simulink model "buffer"  (R2020a)
settings: Solver=VariableStepAuto  StartTime=0.0  StopTime=10.0  RelTol=1e-3
settings Model: Creator=ysz  LastModifiedBy=ysz

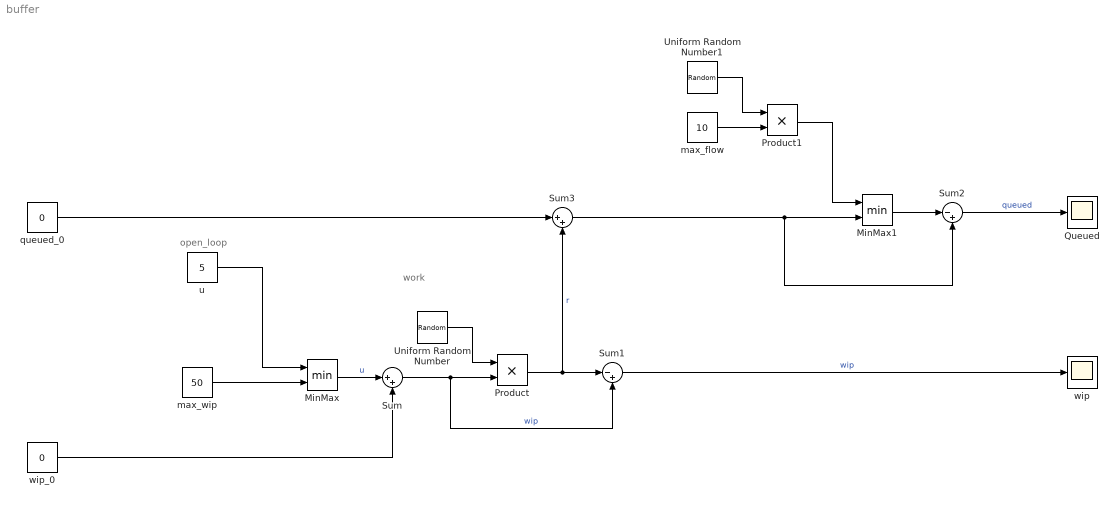
== system buffer ==
  note: open_loop
  note: work
  MinMax : MinMax  Inputs=2
  MinMax1 : MinMax  Inputs=2
  Product : Product
  Product1 : Product
  Queued : Scope
  Sum : Sum  Inputs=|++
  Sum1 : Sum  Inputs=|-+
  Sum2 : Sum  Inputs=|-+
  Sum3 : Sum  Inputs=|++
  Uniform Random Number : UniformRandomNumber  Minimum=0  SampleTime=0.1
  Uniform Random Number1 : UniformRandomNumber  Minimum=0  Seed=10  SampleTime=0.1
  max_flow : Constant  Value=10
  max_wip : Constant  Value=50
  queued_0 : Constant  Value=0
  u : Constant  Value=5
  wip : Scope
  wip_0 : Constant  Value=0
  wires:
  u/1 -> MinMax/1
  max_wip/1 -> MinMax/2
  MinMax/1 -> Sum/1  "u"
  wip_0/1 -> Sum/2
  Uniform Random Number/1 -> Product/1
  Sum/1 -> Sum1/2, Product/2  "wip"
  Product/1 -> Sum3/2, Sum1/1  "r"
  Sum1/1 -> wip/1  "wip"
  max_flow/1 -> Product1/2
  Uniform Random Number1/1 -> Product1/1
  Product1/1 -> MinMax1/1
  Sum3/1 -> Sum2/2, MinMax1/2
  MinMax1/1 -> Sum2/1
  Sum2/1 -> Queued/1  "queued"
  queued_0/1 -> Sum3/1
